simulink model "pmSyn_m_1_21"  (R2021b)
settings: Solver=FixedStepAuto  StartTime=0.0  StopTime=20  FixedStep=Ts  RelTol=1e-3
values from neighbouring files (symbols this model uses):
  clarke = 2/3*[1 -0.5 -0.5;0 sqrt(3)/2 -sqrt(3)/2]    [param_pmsm.m]
  fc = 5000    [param_pmsm.m]
  inv_clarke = [1 -0.5 -0.5;0 sqrt(3)/2 -sqrt(3)/2]'    [param_pmsm.m]
  Ismax = 5    [param_pmsm.m]
  J = 0.01    [param_pmsm.m]    (also in parameters_brushless_DC.m)
  Ls = 0.1    [param_pmsm.m]
  P = 2    [param_pmsm.m]
  psi_PM = 0.6    [param_pmsm.m]
  Rs = 5    [param_pmsm.m]
  TnI = T2    (= 0.02)    [param_pmsm.m]
  TnN = 4*TI    (= 0.0016)    [param_pmsm.m]
  Udc = 565    [param_pmsm.m]
  VrI = T2/(2*V1*V2*T1)    (= 0.884955752212)    [param_pmsm.m]
  VrN = 1/(2*VI*VII*TI)    (= 13.8888888889)    [param_pmsm.m]
libraries: simulink x1
settings Model: Creator=student  LastModifiedBy=ganesh
settings DebuggingCC: UnconnectedInputMsg=none  UnconnectedOutputMsg=none  UnconnectedLineMsg=none
settings RTWCC: DLArmComputeVersion=20.02.1

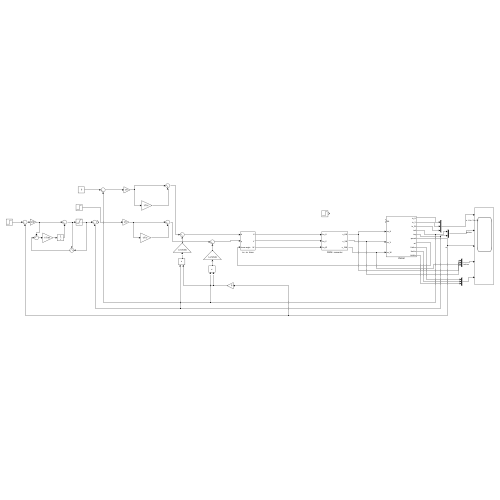
[thumbnail: Simulink's stored preview of the top-level diagram]
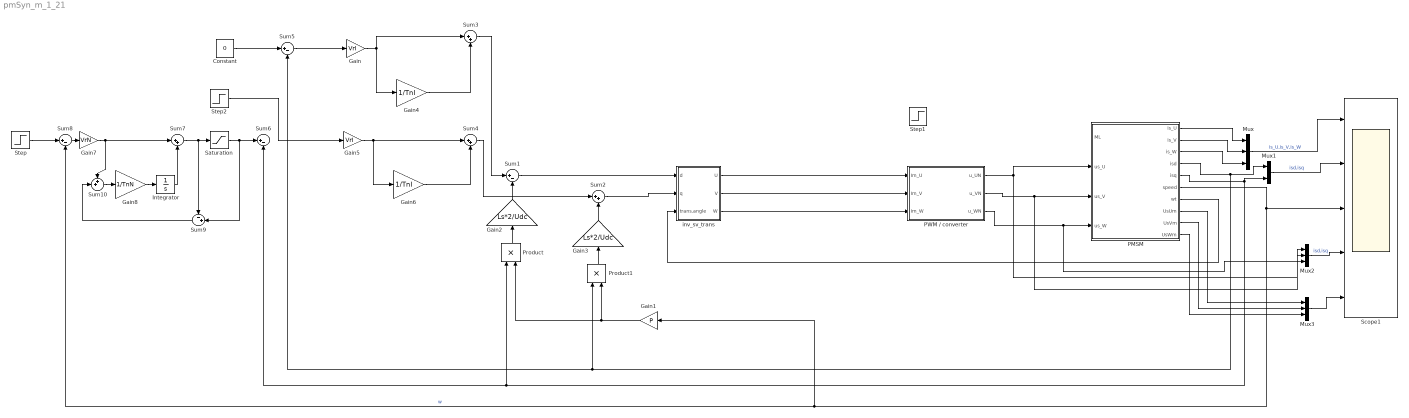
== system pmSyn_m_1_21 ==
  Constant : Constant  Value=0
  Gain : Gain  Gain=VrI
  Gain1 : Gain  Gain=P
  Gain2 : Gain  Gain=Ls*2/Udc
  Gain3 : Gain  Gain=Ls*2/Udc
  Gain4 : Gain  Gain=1/TnI
  Gain5 : Gain  Gain=VrI
  Gain6 : Gain  Gain=1/TnI
  Gain7 : Gain  Gain=VrN
  Gain8 : Gain  Gain=1/TnN
  Integrator : Integrator
  Mux : Mux  Inputs=3
  Mux1 : Mux  Inputs=2
  Mux2 : Mux  Inputs=3
  Mux3 : Mux  Inputs=3
  PMSM : Subsystem
  PWM / converter : Subsystem
  Product : Product
  Product1 : Product
  Saturation : Saturate  UpperLimit=Ismax  LowerLimit=-Ismax
  Scope1 : Scope  NumInputPorts=5
  Step : Step  Time=0.1  After=100  SampleTime=0
  Step1 : Step  Time=0.5  After=5  SampleTime=0
  Step2 : Step  After=10  SampleTime=0
  Sum{1,5..6,8} (4 alike) : Sum  Inputs=|+-
  Sum10 : Sum  Inputs=++|
  Sum{2..4,7} (4 alike) : Sum  Inputs=|++
  Sum9 : Sum  Inputs=-+|
  inv_sv_trans : Subsystem
  wires:
  PMSM/1(is_U) -> Mux/1
  PMSM/2(is_V) -> Mux/2
  PMSM/3(is_W) -> Mux/3
  PMSM/4(isd) -> Sum5/2, Product1/1, Mux1/1
  PMSM/5(isq) -> Sum6/2, Product/1, Mux1/2
  Mux/1 -> Scope1/1  "is_U,is_V,is_W"
  Mux1/1 -> Scope1/2  "isd,isq"
  PMSM/6(speed) -> Sum8/2, Gain1/1, Scope1/3  "w"
  Gain/1 -> Gain4/1, Sum3/1
  Gain4/1 -> Sum3/2
  Gain6/1 -> Sum4/2
  Gain5/1 -> Sum4/1, Gain6/1
  Sum5/1 -> Gain/1
  PMSM/7(wt) -> inv_sv_trans/3(trans.angle)
  Constant/1 -> Sum5/1
  inv_sv_trans/1(U) -> PWM / converter/1(Im_U)
  inv_sv_trans/2(V) -> PWM / converter/2(Im_V)
  inv_sv_trans/3(W) -> PWM / converter/3(Im_W)
  PWM / converter/1(u_UN) -> Mux2/1, PMSM/2(us_U)
  PWM / converter/2(u_VN) -> Mux2/2, PMSM/3(us_V)
  PWM / converter/3(u_WN) -> Mux2/3, PMSM/4(us_W)
  Mux2/1 -> Scope1/4  "isd,isq"
  Gain1/1 -> Product1/2, Product/2
  Sum3/1 -> Sum1/1
  Gain2/1 -> Sum1/2
  Product/1 -> Gain2/1
  Gain3/1 -> Sum2/2
  Product1/1 -> Gain3/1
  Sum4/1 -> Sum2/1
  Sum2/1 -> inv_sv_trans/2(q)
  Sum1/1 -> inv_sv_trans/1(d)
  Gain7/1 -> Sum10/1, Sum7/1
  Sum8/1 -> Gain7/1
  Step/1 -> Sum8/1
  Sum7/1 -> Sum9/1, Saturation/1
  Saturation/1 -> Sum9/2, Sum6/1
  Gain8/1 -> Integrator/1
  Integrator/1 -> Sum7/2
  Sum9/1 -> Sum10/2
  Sum10/1 -> Gain8/1
  PMSM/8(UsUm) -> Mux3/1
  PMSM/9(UsVm) -> Mux3/2
  PMSM/10(UsWm) -> Mux3/3
  Mux3/1 -> Scope1/5
  Step2/1 -> Gain5/1

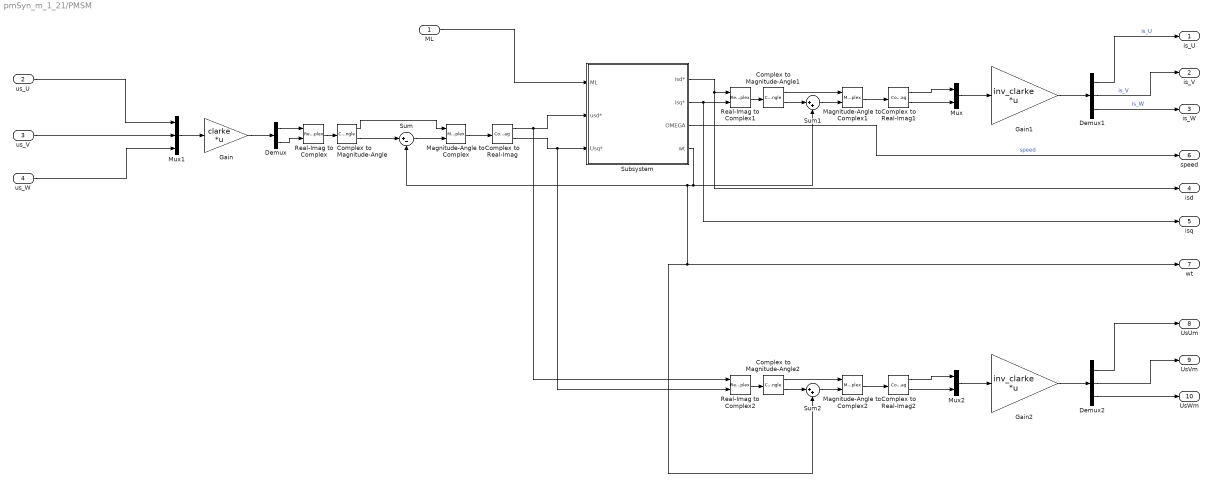
== system pmSyn_m_1_21/PMSM ==
  ML : Inport
  us_U : Inport  Port=2
  us_V : Inport  Port=3
  us_W : Inport  Port=4
  Complex to Magnitude-Angle : ComplexToMagnitudeAngle
  Complex to Magnitude-Angle1 : ComplexToMagnitudeAngle
  Complex to Magnitude-Angle2 : ComplexToMagnitudeAngle
  Complex to Real-Imag : ComplexToRealImag
  Complex to Real-Imag1 : ComplexToRealImag
  Complex to Real-Imag2 : ComplexToRealImag
  Demux : Demux  Outputs=2
  Demux1 : Demux  Outputs=3
  Demux2 : Demux  Outputs=3
  Gain : Gain  Gain=clarke  Multiplication=Matrix(K*u)
  Gain1 : Gain  Gain=inv_clarke  Multiplication=Matrix(K*u)
  Gain2 : Gain  Gain=inv_clarke  Multiplication=Matrix(K*u)
  Magnitude-Angle to Complex : MagnitudeAngleToComplex
  Magnitude-Angle to Complex1 : MagnitudeAngleToComplex
  Magnitude-Angle to Complex2 : MagnitudeAngleToComplex
  Mux : Mux  Inputs=2
  Mux1 : Mux  Inputs=3
  Mux2 : Mux  Inputs=2
  Real-Imag to Complex : RealImagToComplex
  Real-Imag to Complex1 : RealImagToComplex
  Real-Imag to Complex2 : RealImagToComplex
  Subsystem : Subsystem
  Sum : Sum  Inputs=|+-
  Sum1 : Sum  Inputs=|++
  Sum2 : Sum  Inputs=|++
  is_U : Outport
  is_V : Outport  Port=2
  is_W : Outport  Port=3
  isd : Outport  Port=4
  isq : Outport  Port=5
  speed : Outport  Port=6
  wt : Outport  Port=7
  UsUm : Outport  Port=8
  UsVm : Outport  Port=9
  UsWm : Outport  Port=10
  wires:
  Complex to Real-Imag1/1 -> Mux/1
  Gain1/1 -> Demux1/1
  us_U/1 -> Mux1/1
  Mux/1 -> Gain1/1
  Subsystem/1(isd*) -> isd/1, Real-Imag to Complex1/1
  Subsystem/2(isq*) -> Real-Imag to Complex1/2, isq/1
  Demux1/3 -> is_W/1  "is_W"
  Real-Imag to Complex/1 -> Complex to Magnitude-Angle/1
  Magnitude-Angle to Complex/1 -> Complex to Real-Imag/1
  Mux1/1 -> Gain/1
  Sum1/1 -> Magnitude-Angle to Complex1/2
  Demux/2 -> Real-Imag to Complex/2
  Complex to Magnitude-Angle/2 -> Sum/1
  Demux/1 -> Real-Imag to Complex/1
  Gain/1 -> Demux/1
  Complex to Magnitude-Angle1/1 -> Magnitude-Angle to Complex1/1
  Complex to Magnitude-Angle/1 -> Magnitude-Angle to Complex/1
  Complex to Real-Imag1/2 -> Mux/2
  ML/1 -> Subsystem/1(ML)
  Real-Imag to Complex1/1 -> Complex to Magnitude-Angle1/1
  us_V/1 -> Mux1/2
  Sum/1 -> Magnitude-Angle to Complex/2
  Demux1/2 -> is_V/1  "is_V"
  Magnitude-Angle to Complex1/1 -> Complex to Real-Imag1/1
  Complex to Magnitude-Angle1/2 -> Sum1/1
  Demux1/1 -> is_U/1  "is_U"
  us_W/1 -> Mux1/3
  Subsystem/3(OMEGA) -> speed/1  "speed"
  Demux2/1 -> UsUm/1
  Complex to Magnitude-Angle2/2 -> Sum2/1
  Magnitude-Angle to Complex2/1 -> Complex to Real-Imag2/1
  Demux2/2 -> UsVm/1
  Real-Imag to Complex2/1 -> Complex to Magnitude-Angle2/1
  Complex to Real-Imag2/2 -> Mux2/2
  Complex to Magnitude-Angle2/1 -> Magnitude-Angle to Complex2/1
  Sum2/1 -> Magnitude-Angle to Complex2/2
  Demux2/3 -> UsWm/1
  Complex to Real-Imag/2 -> Real-Imag to Complex2/2, Subsystem/3(Usq*)
  Complex to Real-Imag/1 -> Real-Imag to Complex2/1, Subsystem/2(usd*)
  Mux2/1 -> Gain2/1
  Gain2/1 -> Demux2/1
  Complex to Real-Imag2/1 -> Mux2/1
  Subsystem/4(wt) -> Sum1/2, wt/1, Sum2/2, Sum/2

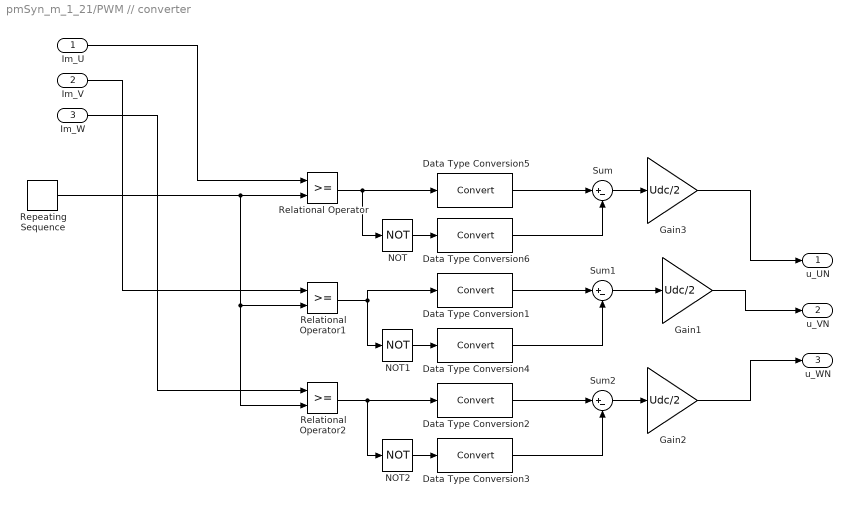
== system pmSyn_m_1_21/PWM // converter ==
  Im_U : Inport
  Im_V : Inport  Port=2
  Im_W : Inport  Port=3
  Data Type Conversion{1..6} (6 alike) : DataTypeConversion
  Gain1 : Gain  Gain=Udc/2
  Gain2 : Gain  Gain=Udc/2
  Gain3 : Gain  Gain=Udc/2
  NOT : Logic  Operator=NOT  IconShape=distinctive  AllPortsSameDT=off  OutDataTypeStr=boolean
  NOT1 : Logic  Operator=NOT  IconShape=distinctive  AllPortsSameDT=off  OutDataTypeStr=boolean
  NOT2 : Logic  Operator=NOT  IconShape=distinctive  AllPortsSameDT=off  OutDataTypeStr=boolean
  Relational Operator : RelationalOperator  OutDataTypeStr=boolean  RndMeth=Simplest
  Relational Operator1 : RelationalOperator  OutDataTypeStr=boolean  RndMeth=Simplest
  Relational Operator2 : RelationalOperator  OutDataTypeStr=boolean  RndMeth=Simplest
  Repeating Sequence : simulink/Sources/Repeating Sequence  rep_seq_t=[0 1/fc]  rep_seq_y=[-1 1]
  Sum : Sum  Inputs=|+-
  Sum1 : Sum  Inputs=|+-
  Sum2 : Sum  Inputs=|+-
  u_UN : Outport
  u_VN : Outport  Port=2
  u_WN : Outport  Port=3
  wires:
  Gain3/1 -> u_UN/1
  Gain1/1 -> u_VN/1
  Relational Operator2/1 -> Data Type Conversion2/1, NOT2/1
  Relational Operator1/1 -> Data Type Conversion1/1, NOT1/1
  Relational Operator/1 -> Data Type Conversion5/1, NOT/1
  Im_V/1 -> Relational Operator1/1
  Repeating Sequence/1 -> Relational Operator/2, Relational Operator1/2, Relational Operator2/2
  Sum/1 -> Gain3/1
  Sum1/1 -> Gain1/1
  Im_U/1 -> Relational Operator/1
  Im_W/1 -> Relational Operator2/1
  Gain2/1 -> u_WN/1
  Sum2/1 -> Gain2/1
  Data Type Conversion2/1 -> Sum2/1
  NOT2/1 -> Data Type Conversion3/1
  Data Type Conversion3/1 -> Sum2/2
  NOT1/1 -> Data Type Conversion4/1
  Data Type Conversion4/1 -> Sum1/2
  Data Type Conversion1/1 -> Sum1/1
  NOT/1 -> Data Type Conversion6/1
  Data Type Conversion5/1 -> Sum/1
  Data Type Conversion6/1 -> Sum/2

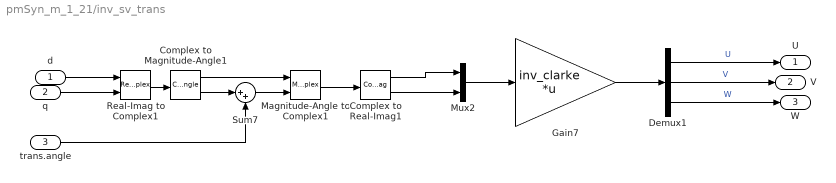
== system pmSyn_m_1_21/inv_sv_trans ==
  d : Inport
  q : Inport  Port=2
  trans.angle : Inport  Port=3
  Complex to Magnitude-Angle1 : ComplexToMagnitudeAngle
  Complex to Real-Imag1 : ComplexToRealImag
  Demux1 : Demux  Outputs=3
  Gain7 : Gain  Gain=inv_clarke  Multiplication=Matrix(K*u)
  Magnitude-Angle to Complex1 : MagnitudeAngleToComplex
  Mux2 : Mux  Inputs=2
  Real-Imag to Complex1 : RealImagToComplex
  Sum7 : Sum  Inputs=|++
  U : Outport
  V : Outport  Port=2
  W : Outport  Port=3
  wires:
  q/1 -> Real-Imag to Complex1/2
  Sum7/1 -> Magnitude-Angle to Complex1/2
  Complex to Magnitude-Angle1/2 -> Sum7/1
  Complex to Real-Imag1/2 -> Mux2/2
  Complex to Magnitude-Angle1/1 -> Magnitude-Angle to Complex1/1
  Magnitude-Angle to Complex1/1 -> Complex to Real-Imag1/1
  Real-Imag to Complex1/1 -> Complex to Magnitude-Angle1/1
  Complex to Real-Imag1/1 -> Mux2/1
  Mux2/1 -> Gain7/1
  Gain7/1 -> Demux1/1
  trans.angle/1 -> Sum7/2
  Demux1/2 -> V/1  "V"
  d/1 -> Real-Imag to Complex1/1
  Demux1/1 -> U/1  "U"
  Demux1/3 -> W/1  "W"

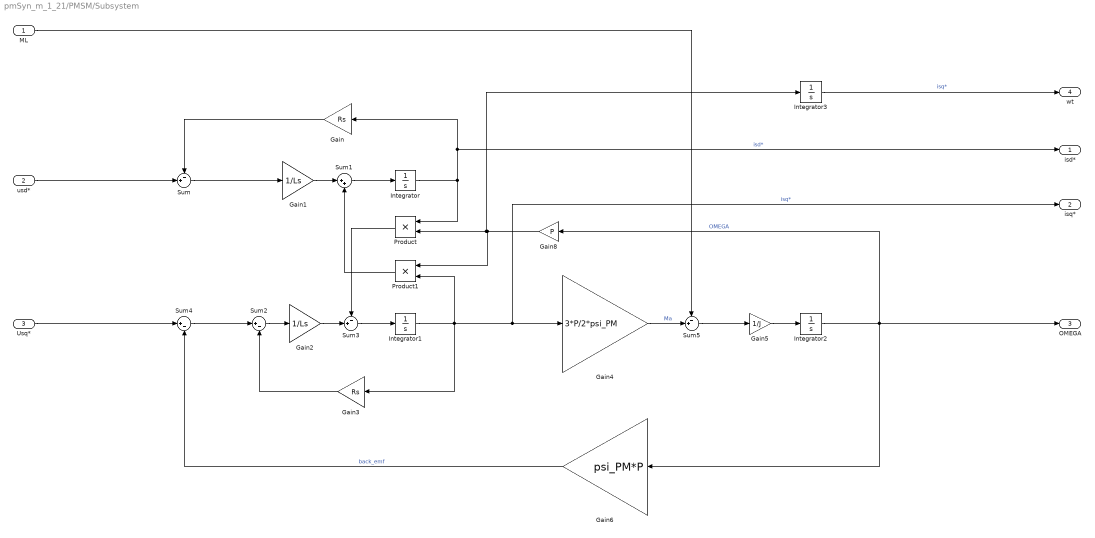
== system pmSyn_m_1_21/PMSM/Subsystem ==
  ML : Inport
  usd* : Inport  Port=2
  Usq* : Inport  Port=3
  Gain : Gain  Gain=Rs
  Gain1 : Gain  Gain=1/Ls
  Gain2 : Gain  Gain=1/Ls
  Gain3 : Gain  Gain=Rs
  Gain4 : Gain  Gain=3*P/2*psi_PM
  Gain5 : Gain  Gain=1/J
  Gain6 : Gain  Gain=psi_PM*P
  Gain8 : Gain  Gain=P
  Integrator{,1..3} (4 alike) : Integrator
  Product : Product
  Product1 : Product
  Sum : Sum  Inputs=-+|
  Sum1 : Sum  Inputs=|++
  Sum2 : Sum  Inputs=|+-
  Sum3 : Sum  Inputs=-+|
  Sum4 : Sum  Inputs=|+-
  Sum5 : Sum  Inputs=-+|
  isd* : Outport
  isq* : Outport  Port=2
  OMEGA : Outport  Port=3
  wt : Outport  Port=4
  wires:
  Gain2/1 -> Sum3/2
  Gain1/1 -> Sum1/1
  Sum2/1 -> Gain2/1
  Integrator/1 -> isd*/1, Gain/1, Product/1  "isd*"
  Gain5/1 -> Integrator2/1
  Sum1/1 -> Integrator/1
  Sum5/1 -> Gain5/1
  Integrator1/1 -> Product1/2, isq*/1, Gain4/1, Gain3/1  "isq*"
  Product1/1 -> Sum1/2
  Sum3/1 -> Integrator1/1
  usd*/1 -> Sum/2
  Sum/1 -> Gain1/1
  Product/1 -> Sum3/1
  Gain/1 -> Sum/1
  Sum4/1 -> Sum2/1
  Gain3/1 -> Sum2/2
  Gain4/1 -> Sum5/2  "Ma"
  Integrator2/1 -> Gain8/1, OMEGA/1, Gain6/1  "OMEGA"
  Gain6/1 -> Sum4/2  "back_emf"
  Gain8/1 -> Product1/1, Integrator3/1, Product/2
  Usq*/1 -> Sum4/1
  ML/1 -> Sum5/1
  Integrator3/1 -> wt/1  "isq*"
